simulink library "propul"  (R2022b)
settings: Solver=VariableStepAuto  StartTime=0.0  StopTime=10.0  RelTol=1e-3
undefined symbols (not defined in the file): alfaf_deg, nrho, nv, rho_reference_kgpm3, Tmax, V_reference_mps, xf_m, zf_m
settings Model: Creator=Dell  LastModifiedBy=Dell

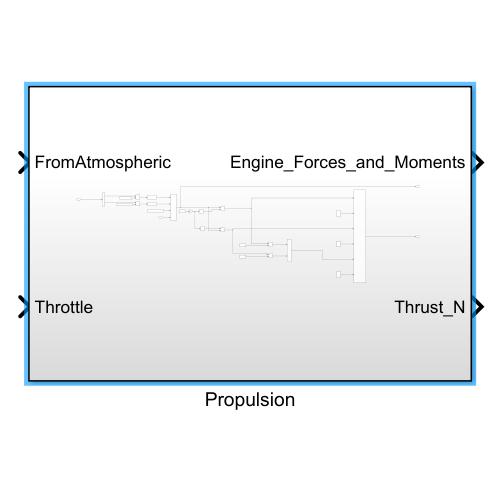
[thumbnail: Simulink's stored preview of the top-level diagram]
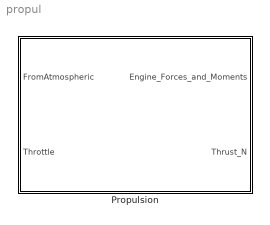
== system propul ==
  Propulsion : Subsystem

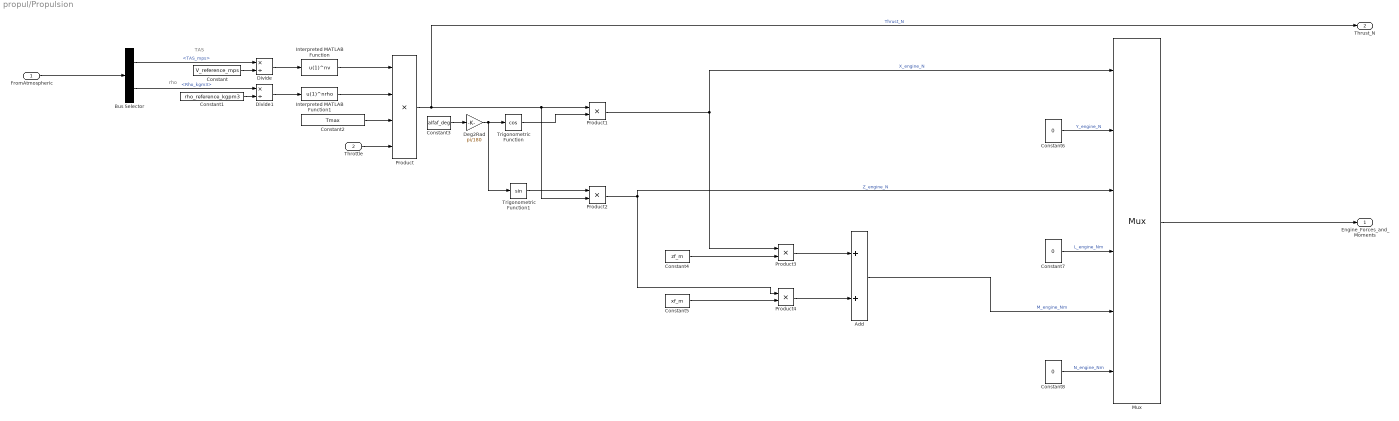
== system propul/Propulsion ==
  note: TAS
  note: rho
  FromAtmospheric : Inport
  Throttle : Inport  Port=2
  Add : Sum
  Bus Selector : BusSelector  OutputSignals=TAS_mps,Rho_kgm3
  Constant : Constant  Value=V_reference_mps
  Constant1 : Constant  Value=rho_reference_kgpm3
  Constant2 : Constant  Value=Tmax
  Constant3 : Constant  Value=alfaf_deg
  Constant4 : Constant  Value=zf_m
  Constant5 : Constant  Value=xf_m
  Constant6 : Constant  Value=0
  Constant7 : Constant  Value=0
  Constant8 : Constant  Value=0
  Deg2Rad : Gain  Gain=pi/180
  Divide : Product  Inputs=*/
  Divide1 : Product  Inputs=*/
  Interpreted MATLAB Function : MATLABFcn  MATLABFcn=u(1)^nv
  Interpreted MATLAB Function1 : MATLABFcn  MATLABFcn=u(1)^nrho
  Mux : Mux  Inputs=6
  Product : Product  Inputs=4
  Product{1..4} (4 alike) : Product
  Trigonometric Function : Trigonometry  Operator=cos
  Trigonometric Function1 : Trigonometry
  Engine_Forces_and_Moments : Outport
  Thrust_N : Outport  Port=2
  wires:
  Product3/1 -> Add/1
  Product/1 -> Thrust_N/1, Product2/2, Product1/1  "Thrust_N"
  Bus Selector/1 -> Divide/1  "<TAS_mps>"
  Divide/1 -> Interpreted MATLAB Function/1
  Bus Selector/2 -> Divide1/1  "<Rho_kgm3>"
  Constant/1 -> Divide/2
  Interpreted MATLAB Function1/1 -> Product/2
  FromAtmospheric/1 -> Bus Selector/1
  Interpreted MATLAB Function/1 -> Product/1
  Deg2Rad/1 -> Trigonometric Function1/1, Trigonometric Function/1
  Constant5/1 -> Product4/2
  Constant2/1 -> Product/3
  Throttle/1 -> Product/4
  Product4/1 -> Add/2
  Mux/1 -> Engine_Forces_and_Moments/1
  Constant4/1 -> Product3/2
  Product2/1 -> Mux/3, Product4/1  "Z_engine_N"
  Constant7/1 -> Mux/4  "L_engine_Nm"
  Product1/1 -> Mux/1, Product3/1  "X_engine_N"
  Constant8/1 -> Mux/6  "N_engine_Nm"
  Add/1 -> Mux/5  "M_engine_Nm"
  Trigonometric Function/1 -> Product1/2
  Constant1/1 -> Divide1/2
  Trigonometric Function1/1 -> Product2/1
  Divide1/1 -> Interpreted MATLAB Function1/1
  Constant3/1 -> Deg2Rad/1
  Constant6/1 -> Mux/2  "Y_engine_N"
